simulink model "Casadi_Custom_Driver"  (R2016b)
settings: Solver=FixedStepDiscrete  StartTime=0.0  StopTime=inf  FixedStep=0.01  RelTol=1e-3  EnableMultiTasking=on
undefined symbols (not defined in the file): dimensionsFactor, DiscIntNeverNeededParam, vehicle_name, VehicleRoadInfoStructSize
libraries: simulink x39, SCANeR_API x36
(part 3 of 3)

== system Casadi_Custom_Driver/lateral control/Subsystem1/Enabled Subsystem1 ==
  In1 : Inport
  In2 : Inport  Port=2
  In3 : Inport  Port=3
  In4 : Inport  Port=4
  In5 : Inport  Port=5
  In6 : Inport  Port=6
  In7 : Inport  Port=7
  In8 : Inport  Port=8
  In9 : Inport  Port=9
  Enable : EnablePort
  MATLAB System6 : MATLABSystem  System=casadi_block_MPCtry_5  SimulateUsing=Interpreted execution
      mask Type: casadi_block_MPCtry_5
      mask Display:
      | disp('casadi_block_MPCtry_5');
      | port_label('input',1,'xd_in');
      | port_label('input',2,'yd_in');
      | port_label('input',3,'yawd_in');
      | port_label('input',4,'yaw_in');
      | port_label('input',5,'x_in');
      | port_label('input',6,'y_in');
      | port_label('input',7,'t');
      | port_label('input',8,'r');
      | port_label('input',9,'ex');
      | port_label('output',1,'delta_out');
      | port_label('output',2,'acc_out');
      | port_label('output',3,'break_out');
      | port_label('output',4,'vref');
      | port_label('output',5,'err');
  Out1 : Outport
  Out2 : Outport  Port=2
  Out3 : Outport  Port=3
  Out4 : Outport  Port=4
  Out5 : Outport  Port=5
  wires:
  In8/1 -> MATLAB System6/8
  MATLAB System6/1 -> Out1/1
  MATLAB System6/2 -> Out2/1
  MATLAB System6/3 -> Out3/1
  MATLAB System6/4 -> Out4/1
  MATLAB System6/5 -> Out5/1
  In1/1 -> MATLAB System6/1
  In2/1 -> MATLAB System6/2
  In3/1 -> MATLAB System6/3
  In4/1 -> MATLAB System6/4
  In5/1 -> MATLAB System6/5
  In6/1 -> MATLAB System6/6
  In7/1 -> MATLAB System6/7
  In9/1 -> MATLAB System6/9

== system Casadi_Custom_Driver/lateral control/Subsystem1/Enabled Subsystem2 ==
  In1 : Inport
  In2 : Inport  Port=2
  In3 : Inport  Port=3
  In4 : Inport  Port=4
  In5 : Inport  Port=5
  In6 : Inport  Port=6
  In7 : Inport  Port=7
  In8 : Inport  Port=8
  In9 : Inport  Port=9
  Enable : EnablePort
  MATLAB System : MATLABSystem  System=casadi_block_MPC_left_turn_onthego  SimulateUsing=Interpreted execution
      mask Type: casadi_block_MPC_left_turn_onthego
      mask Display:
      | disp('casadi_block_MPC_left_turn_onthego');
      | port_label('input',1,'xd_in');
      | port_label('input',2,'yd_in');
      | port_label('input',3,'yawd_in');
      | port_label('input',4,'yaw_in');
      | port_label('input',5,'x_in');
      | port_label('input',6,'y_in');
      | port_label('input',7,'t');
      | port_label('input',8,'r');
      | port_label('input',9,'alpha');
      | port_label('output',1,'delta_out');
      | port_label('output',2,'acc_out');
      | port_label('output',3,'break_out');
      | port_label('output',4,'vref');
      | port_label('output',5,'err');
  Out1 : Outport
  Out2 : Outport  Port=2
  Out3 : Outport  Port=3
  Out4 : Outport  Port=4
  Out5 : Outport  Port=5
  wires:
  In1/1 -> MATLAB System/1
  In2/1 -> MATLAB System/2
  In3/1 -> MATLAB System/3
  In4/1 -> MATLAB System/4
  In5/1 -> MATLAB System/5
  In7/1 -> MATLAB System/7
  In6/1 -> MATLAB System/6
  In9/1 -> MATLAB System/9
  In8/1 -> MATLAB System/8
  MATLAB System/1 -> Out1/1
  MATLAB System/2 -> Out2/1
  MATLAB System/3 -> Out3/1
  MATLAB System/4 -> Out4/1
  MATLAB System/5 -> Out5/1

== system Casadi_Custom_Driver/lateral control/Subsystem1/Enabled Subsystem3 ==
  In1 : Inport
  In2 : Inport  Port=2
  In3 : Inport  Port=3
  In4 : Inport  Port=4
  In5 : Inport  Port=5
  In6 : Inport  Port=6
  In7 : Inport  Port=7
  In8 : Inport  Port=8
  In9 : Inport  Port=9
  In10 : Inport  Port=10
  Enable : EnablePort
  MATLAB System : MATLABSystem  System=casadi_block_MPC_LSS_curve_onthego  SimulateUsing=Interpreted execution
      mask Type: casadi_block_MPC_LSS_curve_onthego
      mask Display:
      | disp('casadi_block_MPC_LSS_curve_onthego');
      | port_label('input',1,'xd_in');
      | port_label('input',2,'yd_in');
      | port_label('input',3,'yawd_in');
      | port_label('input',4,'yaw_in');
      | port_label('input',5,'x_in');
      | port_label('input',6,'y_in');
      | port_label('input',7,'t');
      | port_label('input',8,'R');
      | port_label('input',9,'vlat_ref');
      | port_label('input',10,'vlongi_ref');
      | port_label('output',1,'delta_out');
      | port_label('output',2,'acc_out');
      | port_label('output',3,'break_out');
      | port_label('output',4,'vref');
      | port_label('output',5,'err');
  Out1 : Outport
  Out2 : Outport  Port=2
  Out3 : Outport  Port=3
  Out4 : Outport  Port=4
  Out5 : Outport  Port=5
  wires:
  In1/1 -> MATLAB System/1
  In2/1 -> MATLAB System/2
  In3/1 -> MATLAB System/3
  In4/1 -> MATLAB System/4
  In5/1 -> MATLAB System/5
  In7/1 -> MATLAB System/7
  In6/1 -> MATLAB System/6
  MATLAB System/1 -> Out1/1
  MATLAB System/2 -> Out2/1
  MATLAB System/3 -> Out3/1
  MATLAB System/4 -> Out4/1
  MATLAB System/5 -> Out5/1
  In10/1 -> MATLAB System/10
  In9/1 -> MATLAB System/9
  In8/1 -> MATLAB System/8

== system Casadi_Custom_Driver/lateral control/Subsystem1/derivation ==
  note: Bricolage perso - a retester - 09/2019
  In1 : Inport
  Add : Sum  Inputs=+-
  Delay : Delay  DelayLength=10  SampleTime=0.01
  Discrete Derivative : simulink/Discrete/Discrete Derivative  gainval=1.0  ICPrevScaledInput=0.0  OutMin=[]  OutMax=[]  OutDataType=fixdt(1, 16)  OutScaling=2^-10  DoSatur=off
  Manual Switch : ManualSwitch
  Transfer Fcn First Order : simulink/Discrete/Transfer Fcn First Order  Commented=through  PoleZ=0.95  ICPrevOutput=0.0  DoSatur=off
  change_sign : Gain  Commented=through  Gain=-1
  coef : Gain  Gain=10
  Out1 : Outport
  wires:
  change_sign/1 -> Manual Switch/1
  coef/1 -> Transfer Fcn First Order/1
  Delay/1 -> Add/2
  Transfer Fcn First Order/1 -> change_sign/1
  In1/1 -> Discrete Derivative/1, Delay/1, Add/1
  Add/1 -> coef/1
  Discrete Derivative/1 -> Manual Switch/2
  Manual Switch/1 -> Out1/1

== system Casadi_Custom_Driver/lateral control/main lateral block/PI controller ==
  In1 : Inport
  Enable1 : EnablePort  StatesWhenEnabling=reset
  Discrete PID Controller3 : simulink/Continuous/PID Controller  Controller=PI  TimeDomain=Discrete-time  SampleTime=0.01  IntegratorMethod=Forward Euler  FilterMethod=Forward Euler  Form=Parallel  UseFilter=on  ControllerParametersSource=internal  P=1  I=0.4  D=1  N=1  InitialConditionSource=internal  InitialConditionForIntegrator=0  InitialConditionForFilter=0  ExternalReset=none  LimitOutput=off  UpperSaturationLimit=inf  LowerSaturationLimit=-inf  LinearizeAsGain=off  AntiWindupMode=none  Kb=1  TrackingMode=off  Kt=1  PParamMin=[]  PParamMax=[]  IParamMin=[]  IParamMax=[]  DParamMin=[]  DParamMax=[]  NParamMin=[]  NParamMax=[]  KbParamMin=[]  KbParamMax=[]  KtParamMin=[]  KtParamMax=[]  POutMin=[]  POutMax=[]  IOutMin=[]  IOutMax=[]  DOutMin=[]  DOutMax=[]  NOutMin=[]  NOutMax=[]  KbOutMin=[]  KbOutMax=[]  KtOutMin=[]  KtOutMax=[]  IntegratorOutMin=[]  IntegratorOutMax=[]  FilterOutMin=[]  FilterOutMax=[]  SumOutMin=[]  SumOutMax=[]  SumI1OutMin=[]  SumI1OutMax=[]  SumI2OutMin=[]  SumI2OutMax=[]  SumI3OutMin=[]  SumI3OutMax=[]  SumDOutMin=[]  SumDOutMax=[]  SaturationOutMin=[]  SaturationOutMax=[]  IntegratorContinuousStateAttributes=''  IntegratorStateMustResolveToSignalObject=off  IntegratorRTWStateStorageClass=Auto  FilterContinuousStateAttributes=''  FilterStateMustResolveToSignalObject=off  FilterRTWStateStorageClass=Auto  DifferentiatorICPrevScaledInput=0  DifferentiatorOutMin=[]  DifferentiatorOutMax=[]
  Out1 : Outport
  wires:
  Discrete PID Controller3/1 -> Out1/1
  In1/1 -> Discrete PID Controller3/1

== system Casadi_Custom_Driver/lateral control/main lateral block/Saturation ==
  Vh_Speed_kmh : Inport
  Steering_wheel_rad : Inport  Port=2
  Add5 : Sum  Inputs=+-  SampleTime=0.01
  Compare To Constant2 : simulink/Logic and Bit Operations/Compare To Constant  relop===  const=0  OutDataTypeStr=boolean
  Constant1 : Constant  Value=0
  Delay2 : Delay  DelayLength=1
  Gain1 : Gain  Gain=-1
  Mux1 : Mux  Inputs=2
  Saturation Dynamic : simulink/Discontinuities/Saturation Dynamic  OutMin=[]  OutMax=[]  OutDataTypeStr=Inherit: Same as second input  OutDataType=fixdt(1, 16)  OutScaling=2^-10  DoSatur=off
  Saturation acording vehicle speed : Lookup_n-D  NumberOfTableDimensions=1  BreakpointsForDimension1=[0,10,50,100,150]  BreakpointsForDimension1Min=0  BreakpointsForDimension1Max=150  Table=[1.3,1.25,1.1,0.8,0.3]  TableMin=0  TableMax=7.1  ExtrapMethod=Clip  UseLastTableValue=on  SampleTime=0.01  RndMeth=Simplest  InputSameDT=on
      settings: AttributesFormatString=%<Description>
  PID_sat_flag : Outport
  Driver_Action_to_SCANeR_Lat : Outport  Port=2
  wires:
  Gain1/1 -> Saturation Dynamic/3
  Saturation acording vehicle speed/1 -> Saturation Dynamic/1, Gain1/1
  Constant1/1 -> Mux1/2
  Steering_wheel_rad/1 -> Add5/1, Saturation Dynamic/2
  Add5/1 -> Delay2/1
  Compare To Constant2/1 -> PID_sat_flag/1
  Delay2/1 -> Compare To Constant2/1
  Mux1/1 -> Driver_Action_to_SCANeR_Lat/1
  Saturation Dynamic/1 -> Mux1/1, Add5/2
  Vh_Speed_kmh/1 -> Saturation acording vehicle speed/1

== system Casadi_Custom_Driver/lateral control/main lateral block/ShiftToGap ==
  note: z019013 :LAne gap part can be cleaned up
  note: This block allows to always output a required gap in meters, whatever may be the choice of shift type (1= meters / 0= lanes)
  note: z019013 : Added to v7p7p0 : to enable driver to maintian
      | lane center when offset of 0 is used
  Lane_gap_m : Inport
  Shift_Value : Inport  Port=2
  Shift_Type_1Met_0Lan : Inport  Port=3
  Compare To Constant : simulink/Logic and Bit Operations/Compare To Constant  relop=~=  const=0  OutDataTypeStr=boolean
  Constant : Constant
  Constant2 : Constant
  Logical Operator : Logic  Operator=OR  AllPortsSameDT=off  OutDataTypeStr=boolean
  Memory1 : Memory
  Product6 : Product  SampleTime=0.01  RndMeth=Zero
  Relational Operator : RelationalOperator  Operator===  OutDataTypeStr=boolean  RndMeth=Simplest
  Subsystem4 : Subsystem
  Switch1 : Switch  Criteria=u2 > Threshold  Threshold=0.5
  Switch3 : Switch  Criteria=u2 > Threshold  Threshold=0.5
  Lateral_Shift_flag : Outport
  Desired_Gap_offset_m : Outport  Port=2
  wires:
  Shift_Type_1Met_0Lan/1 -> Relational Operator/1, Switch1/2
  Product6/1 -> Switch1/3
  Lane_gap_m/1 -> Subsystem4/1(Lane_Gap_m)
  Switch1/1 -> Desired_Gap_offset_m/1
  Subsystem4/1(Lane_with_m) -> Product6/2
  Switch3/1 -> Logical Operator/1, Memory1/1
  Constant2/1 -> Switch3/1
  Memory1/1 -> Switch3/3
  Shift_Value/1 -> Compare To Constant/1, Switch1/1, Product6/1
  Compare To Constant/1 -> Switch3/2
  Relational Operator/1 -> Logical Operator/2
  Logical Operator/1 -> Lateral_Shift_flag/1
  Constant/1 -> Relational Operator/2

== system Casadi_Custom_Driver/lateral control/main lateral block/Subsystem ==
  Vehicle_Heading_rad : Inport
  Road_Angle_rad : Inport  Port=2
  Add5 : Sum  Inputs=+-  SampleTime=0.01
  Add6 : Sum  SampleTime=0.01
  Compare To Zero1 : simulink/Logic and Bit Operations/Compare To Zero  relop=>  OutDataTypeStr=boolean
  Constant3 : Constant
  Constant4 : Constant  Value=-1
  Product3 : Product  SampleTime=0.01  RndMeth=Zero
  Product4 : Product  SampleTime=0.01  RndMeth=Zero
  Switch1 : Switch  Threshold=0.5
  Trigonometric Function1 : Trigonometry
  Trigonometric Function2 : Trigonometry  Operator=cos
  Trigonometric Function3 : Trigonometry  Operator=cos
  Trigonometric Function4 : Trigonometry
  Vehicle_direction : Outport
  wires:
  Trigonometric Function1/1 -> Product3/1
  Trigonometric Function4/1 -> Product3/2
  Trigonometric Function2/1 -> Product4/1
  Trigonometric Function3/1 -> Product4/2
  Product3/1 -> Add6/1
  Product4/1 -> Add6/2
  Add6/1 -> Compare To Zero1/1
  Compare To Zero1/1 -> Switch1/2
  Constant4/1 -> Switch1/1
  Constant3/1 -> Switch1/3
  Switch1/1 -> Vehicle_direction/1
  Vehicle_Heading_rad/1 -> Add5/1, Trigonometric Function1/1, Trigonometric Function2/1
  Add5/1 -> Trigonometric Function3/1, Trigonometric Function4/1
  Road_Angle_rad/1 -> Add5/2

== system Casadi_Custom_Driver/lateral control/main lateral block/Subsystem1 ==
  Gap_offset_m : Inport
  Time_Gap_offset_s : Inport  Port=2
  Vh_Speed_kmh : Inport  Port=3
  Abs : Abs
  Add7 : Sum  Inputs=+-  SampleTime=0.01
  Constant : Constant  Value=-1
  Detect Change : simulink/Logic and Bit Operations/Detect Change  vinit=0  OutDataTypeStr=boolean
  Detect Change1 : simulink/Logic and Bit Operations/Detect Change  vinit=0  OutDataTypeStr=boolean
  Logical Operator : Logic  Operator=OR  AllPortsSameDT=off  OutDataTypeStr=boolean
  Manual Switch : ManualSwitch
  Product1 : Product  Inputs=*/  SampleTime=0.01  RndMeth=Zero
  Product2 : Product  Inputs=**  SampleTime=0.01  RndMeth=Zero
  Rate Limiter Dynamic : simulink/Discontinuities/Rate Limiter Dynamic
  Saturation : Saturate  UpperLimit=inf  LowerLimit=0
  Switch1 : Switch  Threshold=0.0
  Switch2 : Switch  Threshold=0.0
  Triggered Subsystem1 : Subsystem  TreatAsAtomicUnit=on
  coefficient acording vehicle speed1 : Lookup_n-D  NumberOfTableDimensions=1  BreakpointsForDimension1=[0,20,100,200]  Table=[3,3,1,1]  SampleTime=0.01  RndMeth=Simplest  InputSameDT=on
  lo : Constant  Value=-1
  lo1 : Constant
  Gap_offset_Final_m : Outport
  wires:
  Time_Gap_offset_s/1 -> Detect Change1/1, Add7/1
  coefficient acording vehicle speed1/1 -> Add7/2
  Add7/1 -> Saturation/1
  Vh_Speed_kmh/1 -> coefficient acording vehicle speed1/1
  Saturation/1 -> Product1/2
  [Gap_offset_m] -> Rate Limiter Dynamic/2, Switch1/2, Switch2/2
  lo/1 -> Switch1/1
  Rate Limiter Dynamic/1 -> Gap_offset_Final_m/1
  lo1/1 -> Switch2/3
  Gap_offset_m/1 -> Triggered Subsystem1/1(In1), Manual Switch/2, Abs/1, Detect Change/1
  Detect Change/1 -> Logical Operator/1
  Triggered Subsystem1/1(Out1) -> Manual Switch/1
  Manual Switch/1 -> [Gap_offset_m]
  Abs/1 -> Product1/1
  Product1/1 -> Product2/1, Switch2/1
  Product2/1 -> Switch1/3
  Constant/1 -> Product2/2
  Switch2/1 -> Rate Limiter Dynamic/1
  Switch1/1 -> Rate Limiter Dynamic/3
  Detect Change1/1 -> Logical Operator/2
  Logical Operator/1 -> Triggered Subsystem1/Trigger

== system Casadi_Custom_Driver/lateral control/main lateral block/Subsystem5 ==
  Road_Gap_m : Inport
  Road_Gap_Offset_m : Inport  Port=2
  Add5 : Sum  Inputs=+-  SampleTime=0.01
  Road_Gap_Err_m : Outport
  wires:
  Add5/1 -> Road_Gap_Err_m/1
  Road_Gap_m/1 -> Add5/2
  Road_Gap_Offset_m/1 -> Add5/1

== system Casadi_Custom_Driver/longitudinal control/Speed_Regulation/tolerance_calculation ==
  Cste2 : Constant  Value=vehicle_name  SampleTime=0.01
  Cste4 : Constant  Value=21  SampleTime=0.01
  Cste5 : Constant  Value=0.4  SampleTime=0.01
  Cste6 : Constant  Value=0.1  SampleTime=0.01
  Relational Operator : RelationalOperator  Operator===  OutDataTypeStr=boolean  RndMeth=Simplest
  Switch : Switch  Criteria=u2 > Threshold  Threshold=0.5
  Out1 : Outport
  wires:
  Switch/1 -> Out1/1
  Cste6/1 -> Switch/3
  Cste5/1 -> Switch/1
  Cste2/1 -> Relational Operator/1
  Cste4/1 -> Relational Operator/2
  Relational Operator/1 -> Switch/2

== system Casadi_Custom_Driver/Input_Signals_Management/Subsystem2/Road_Gap_Offset_Calculate1/Triggered Subsystem ==
  In1 : Inport
  Trigger : TriggerPort  VariantControl=Variant
  Out1 : Outport
  wires:
  In1/1 -> Out1/1

== system Casadi_Custom_Driver/lateral control/main lateral block/ShiftToGap/Subsystem4 ==
  Lane_Gap_m : Inport
  Subsystem3 : Subsystem
  Lane_with_m : Outport
  wires:
  Subsystem3/1(Lane_with_m) -> Lane_with_m/1
  Lane_Gap_m/1 -> Subsystem3/1(Lane_Gap_m)

== system Casadi_Custom_Driver/lateral control/main lateral block/Subsystem1/Triggered Subsystem1 ==
  In1 : Inport
  Trigger : TriggerPort  VariantControl=Variant
  Add : Sum
  Constant : Constant  Value=0
  Switch : Switch  Criteria=u2 ~= 0  Threshold=0.0
  Unit Delay : UnitDelay  SampleTime=-1
  Out1 : Outport
  wires:
  Unit Delay/1 -> Add/2
  Add/1 -> Switch/1, Switch/2, Unit Delay/1
  In1/1 -> Add/1
  Switch/1 -> Out1/1
  Constant/1 -> Switch/3

== system Casadi_Custom_Driver/lateral control/main lateral block/ShiftToGap/Subsystem4/Subsystem3 ==
  Lane_Gap_m : Inport
  Abs : Abs
  Abs1 : Abs
  Compare To Constant1 : simulink/Logic and Bit Operations/Compare To Constant  relop=>  const=1  OutDataTypeStr=boolean
  Compare To Zero : simulink/Logic and Bit Operations/Compare To Zero  relop=<  OutDataTypeStr=boolean
  Constant1 : Constant  Value=3.5
  Constant2 : Constant
  Logical Operator : Logic  AllPortsSameDT=off  OutDataTypeStr=boolean
  Logical Operator1 : Logic  Operator=NOT  AllPortsSameDT=off  OutDataTypeStr=boolean
  Memory : Memory
  Memory1 : Memory
  Product11 : Product
  Switch1 : Switch  Criteria=u2 > Threshold  Threshold=0.5
  Switch2 : Switch  Criteria=u2 > Threshold  Threshold=0.5
  Switch3 : Switch  Criteria=u2 > Threshold  Threshold=0.5
  Unit Delay : UnitDelay  SampleTime=-1
  g : Gain  Gain=2
  Lane_with_m : Outport
  wires:
  Switch3/1 -> Switch1/2, Memory1/1, Logical Operator1/1
  Lane_Gap_m/1 -> Unit Delay/1, Abs/1, Product11/1
  Constant2/1 -> Switch3/1
  Memory1/1 -> Switch3/3
  Compare To Constant1/1 -> Logical Operator/1
  Logical Operator/1 -> Switch3/2
  Switch1/1 -> g/1, Memory/1
  Memory/1 -> Switch1/1
  Product11/1 -> Compare To Zero/1
  Unit Delay/1 -> Product11/2, Switch1/3
  Compare To Zero/1 -> Logical Operator/2
  Abs/1 -> Compare To Constant1/1
  Switch2/1 -> Lane_with_m/1
  g/1 -> Abs1/1
  Constant1/1 -> Switch2/1
  Logical Operator1/1 -> Switch2/2
  Abs1/1 -> Switch2/3

== stateflow chart Casadi_Custom_Driver/longitudinal control/Accel_Regulation/Chart1 ==
  state Accel_Control/
    state Control_Off/
      accel_order= 0;
      brake_order= 0;
      accel_dyn= 0;
      brake_dyn= 0;
      int_epsilon = 0;
      Gear=10;
    state Controller/
      limit_accel = 1/kp_acc;
      limit_brake = 1/kp_brk;
      state Acceleration_regulation/
        state accel/
          control_state = 2;
          accel_order=1;
          brake_order= 0;
          accel_dyn=  kp_acc*epsilon + ki_acc*int_epsilon;
          brake_dyn= 0;
          Gear=10;
        (junction 59) -> accel [order 1] : [abs(epsilon) < limit_accel & control_state == 2]
            | {int_epsilon = int_epsilon + step_size*epsilon;}
        (junction 59) -> accel [order 2] : {int_epsilon = 0;}
      state Brake_regulation/
        state brake/
          control_state = 1;
          accel_order=0;
          brake_order=1;
          accel_dyn= 0;
          brake_dyn=  kp_brk*epsilon + ki_brk*int_epsilon;
          Gear=10;
        (junction 101) -> brake [order 1] : [abs(epsilon) < limit_brake & control_state == 1]
            | {int_epsilon = int_epsilon + step_size*epsilon;}
        (junction 101) -> brake [order 2] : {int_epsilon = 0;}
      accel -> (junction 56)
      brake -> (junction 56)
      (junction 56) -> (junction 59) [order 1] : [Accel_SP >= 0]
          | {epsilon =Accel_SP-Accel_Actual;}
      (junction 56) -> (junction 101) [order 2] : {epsilon =Accel_Actual-Accel_SP;}
    (default) -> (junction 55)
    (junction 55) -> Control_Off [order 1] : [Accel_control_on == 0]
    Control_Off -> (junction 55)
    Controller -> (junction 55) : [Accel_control_on == 0]
    (junction 55) -> (junction 56) [order 2] : {control_state = 0;}
  data: Accel_Actual input double; Accel_SP input double; Accel_control_on input double; accel_order output double; accel_dyn output double; brake_order output double; brake_dyn output double; kp_acc input double; ki_acc input double; kp_brk input double; ki_brk input double; step_size input double; limit_accel local double; limit_brake local double; epsilon output double; int_epsilon output double; control_state output double; Gear output double

== stateflow chart Casadi_Custom_Driver/longitudinal control/Speed_Regulation/Chart1 ==
  state Speed_Control/
    state Control_Off/
      accel = 0;
      brake = 0;
      int_epsilon = 0;
      Gear=3;
    state Controller/
      limit_accel = 1/kp_acc;
      limit_brake = 1/kp_brk;
      state normal_regulation/
        state normal_accel/
          control_state = 2;
          accel = -kp_acc*epsilon - ki_acc*int_epsilon;
          brake = 0;
          Gear_d = Gear;
        state normal_brake/
          control_state = 1;
          brake = kp_brk*epsilon + ki_brk*int_epsilon;
          accel = 0;
          Gear_d = Gear;
        (junction 58) -> (junction 59) [order 1] : [epsilon <= tolerance]
        (junction 58) -> (junction 57) [order 2]
        (junction 59) -> Speed_Control.Controller.normal_regulation.normal_accel [order 1] : [abs(epsilon) < limit_accel & control_state == 2]
            | {int_epsilon = int_epsilon + step_size*epsilon;}
        (junction 59) -> Speed_Control.Controller.normal_regulation.normal_accel [order 2] : {int_epsilon = 0;}
        (junction 57) -> Speed_Control.Controller.normal_regulation.normal_brake [order 1] : [abs(epsilon) < limit_brake & control_state == 1]
            | {int_epsilon = int_epsilon + step_size*epsilon;}
        (junction 57) -> Speed_Control.Controller.normal_regulation.normal_brake [order 2] : {int_epsilon = 0;}
        Speed_Control.Controller.normal_regulation.normal_brake -> (junction 69)
        Speed_Control.Controller.normal_regulation.normal_accel -> (junction 69)
      state reverse_regulation1/
        state normal_accel/
          control_state = 2;
          accel = -kp_acc*epsilon - ki_acc*int_epsilon;
          brake = 0;
          Gear_d = Gear;
        state normal_brake/
          control_state = 1;
          brake = kp_brk*epsilon + ki_brk*int_epsilon;
          accel = 0;
          Gear_d = Gear;
        (junction 123) -> (junction 124) [order 1] : [epsilon <=-0.1]
        (junction 123) -> (junction 125) [order 2]
        (junction 124) -> Speed_Control.Controller.reverse_regulation1.normal_accel [order 1] : [abs(epsilon) < limit_accel & control_state == 2]
            | {int_epsilon = int_epsilon + step_size*epsilon;}
        (junction 124) -> Speed_Control.Controller.reverse_regulation1.normal_accel [order 2] : {int_epsilon = 0;}
        (junction 125) -> Speed_Control.Controller.reverse_regulation1.normal_brake [order 1] : [abs(epsilon) < limit_brake & control_state == 1]
            | {int_epsilon = int_epsilon + step_size*epsilon;}
        (junction 125) -> Speed_Control.Controller.reverse_regulation1.normal_brake [order 2] : {int_epsilon = 0;}
        Speed_Control.Controller.reverse_regulation1.normal_brake -> (junction 126)
        Speed_Control.Controller.reverse_regulation1.normal_accel -> (junction 126)
      (junction 56) -> (junction 99) [order 1] : [setpoint< 0]
          | {epsilon =- speed+setpoint;}
      (junction 56) -> (junction 62) [order 2] : {epsilon = speed-setpoint;}
      (junction 62) -> (junction 58) : {Gear =10;}
      (junction 69) -> (junction 56)
      (junction 126) -> (junction 56)
      (junction 99) -> (junction 123) : {Gear =2;}
    (default) -> (junction 55)
    (junction 55) -> Control_Off [order 1] : [speed_control_on == 0]
    Control_Off -> (junction 55)
    Controller -> (junction 55) : [speed_control_on == 0]
    (junction 55) -> (junction 56) [order 2] : {control_state = 0;}
  data: speed input double; setpoint input double; speed_control_on input double; accel output double; brake output double; kp_acc input double; ki_acc input double; kp_brk input double; ki_brk input double; step_size input double; limit_accel local double; limit_brake local double; epsilon output double; int_epsilon output double; control_state output double; Gear_d output double; Gear local double; tolerance input double

== matlab function Casadi_Custom_Driver/longitudinal control/Speed_Regulation/MATLAB Function ==
  data: vehicle_name input; Kp_Accl output; Ki_Accl output; Intended_Vehicle_Speed_kmph input
function [Kp_Accl, Ki_Accl]= fcn(vehicle_name,Intended_Vehicle_Speed_kmph)
% This function calculates the Kp_Accl and Ki_Accl
% Following are the vehicle models to be used for simulation
% Vehicle_name:
% 0 = HHN
% 1 = BCB
% 2 = FFK
% 3 = KFKL1
% 4 = KFKL2
% 5 = KFKL1_VODM_CD04
% 6= KFKL1_VODM_CD05
% 7 = KFKL1_VODM_CD06
% 8 = FFKL1_VODM_CD06
% 9 = FFKL1_MMAC_CD06
% 10 = FFKL2_MMAC_CD06
% 11 = KFKL2_MMAC_CD06
% 12 = XDD

if (vehicle_name == 0)
    Kp_Accl = 0.3;
    Ki_Accl = 0.05;
elseif (vehicle_name == 1)
    Kp_Accl = 0.3;
    Ki_Accl = 0.05;
elseif (vehicle_name == 2)
    Kp_Accl = 0.1;
    Ki_Accl = 0.02;
elseif (vehicle_name == 3)
    Kp_Accl = 0.3;
    Ki_Accl = 0.02;
elseif (vehicle_name == 4)
    Kp_Accl = 0.3;
    Ki_Accl = 0.02;
elseif (vehicle_name == 5)
    Kp_Accl = 0.3;
    Ki_Accl = 0.02;
elseif (vehicle_name == 6)
    Kp_Accl = 0.3;
    Ki_Accl = 0.02;
elseif (vehicle_name == 7)
    Kp_Accl = 0.3;
    Ki_Accl = 0.02;
elseif (vehicle_name == 8)
    Kp_Accl = 0.3;
    Ki_Accl = 0.02;
elseif (vehicle_name == 9)
    Kp_Accl = 0.3;
    Ki_Accl = 0.02;
elseif (vehicle_name == 10)
    Kp_Accl = 0.3;
    Ki_Accl = 0.02;
elseif (vehicle_name == 11)
    Kp_Accl = 0.3;
    Ki_Accl = 0.02;
elseif (vehicle_name == 17)% HCB 60kwh
    if Intended_Vehicle_Speed_kmph >= 60
        Kp_Accl = 0.3; %0.1
        Ki_Accl = 0.05;%0.01
    else
        Kp_Accl = 0.1; %0.1
        Ki_Accl = 0.01;%0.01
    end
elseif (vehicle_name == 13) || (vehicle_name == 15) % BCB
    Kp_Accl =0.3;
    Ki_Accl = 0.05;
elseif (vehicle_name == 18) || (vehicle_name == 14) || (vehicle_name == 12)% XDD vehicle
    Kp_Accl = 0.3;
    Ki_Accl = 0.05;
elseif (vehicle_name == 19)% BCB 40kwh Correl
    if Intended_Vehicle_Speed_kmph >= 50
        Kp_Accl = 1;
        Ki_Accl = 0.1;
    else
        Kp_Accl = 0.1; %0.1
        Ki_Accl = 0.01;%0.01
    end
elseif (vehicle_name == 16) % HHN Correl
    if Intended_Vehicle_Speed_kmph >= 15
        Kp_Accl = 0.3;
        Ki_Accl = 0.05;
    elseif Intended_Vehicle_Speed_kmph < 7
        Kp_Accl = 0.3;
        Ki_Accl = 0.05;
    else
        Kp_Accl = 0.009;
        Ki_Accl = 0.00032;
    end
elseif (vehicle_name == 20) % Echo
    Kp_Accl = 0.3;
    Ki_Accl = 0.05;
elseif (vehicle_name == 21) % Torque Management
    Kp_Accl = 0.0012;
    Ki_Accl = 0.0012;
else  % Other vehicles
    if Intended_Vehicle_Speed_kmph >= 15
        Kp_Accl = 0.3;
        Ki_Accl = 0.05;
    else
        Kp_Accl = 0.009;
        Ki_Accl = 0.00032;
    end
end

== stateflow chart Casadi_Custom_Driver/driver manager/Chart ==
  state Variablesetting
    entry:
    Driver_Action_to_SCANeR_Long;
    Driver_Action_to_SCANeR_Lat;
    Null_longitudinal;
    Null_lateral;
    manual_acc_brk;
    manual_acc_brk_val;
    APK_steer_rad;
    APK_steer_rad_val;
  state driverstatus0
    entry:
    longitudinal = Null_longitudinal;
    lateral = Null_lateral;
    if APK_steer_rad_val > 0
    lateral = APK_steer_rad;
    end
    if manual_acc_brk_val >0
    longitudinal = manual_acc_brk;
    end
  state driverstatus3
    entry:
    longitudinal = Driver_Action_to_SCANeR_Long;
    lateral = Null_lateral;
    if APK_steer_rad_val > 0
    lateral = APK_steer_rad;
    end
    if manual_acc_brk_val > 0
    longitudinal = manual_acc_brk;
    end
  state driverstatus2
    entry:
    longitudinal = Null_longitudinal;
    lateral = Driver_Action_to_SCANeR_Lat;
    if APK_steer_rad_val > 0
    lateral = APK_steer_rad;
    end
    if manual_acc_brk_val > 0
    longitudinal = manual_acc_brk;
    end
  state driverstatus1
    entry:
    longitudinal = Driver_Action_to_SCANeR_Long;
    lateral = Driver_Action_to_SCANeR_Lat;
    if APK_steer_rad_val > 0
    lateral = APK_steer_rad;
    end
    if manual_acc_brk_val > 0
    longitudinal = manual_acc_brk;
    end
  state driverstatus4
    entry:
    longitudinal = Temp_longitudinal_GLOSA;
    lateral = Temp_lateral_GLOSA;
    if APK_steer_rad_val > 0
    lateral = APK_steer_rad;
    end
    if manual_acc_brk_val > 0
    longitudinal = manual_acc_brk;
    end
  (default) -> Variablesetting
  Variablesetting -> (junction 29)
  driverstatus3 -> (junction 29)
  driverstatus0 -> (junction 29)
  (junction 29) -> driverstatus3 [order 5] : [Driver_status == 3]
  (junction 29) -> driverstatus0 [order 1] : [Driver_status == 0]
  (junction 29) -> driverstatus1 [order 2] : [Driver_status == 1 || Driver_status > 4]
  (junction 29) -> driverstatus2 [order 4] : [Driver_status == 2]
  driverstatus4 -> (junction 29)
  (junction 29) -> driverstatus4 [order 3] : [Driver_status == 4]
  driverstatus1 -> (junction 29)
  driverstatus2 -> (junction 29)
  data: Driver_Action_to_SCANeR_Long input; Driver_Action_to_SCANeR_Lat input; Null_longitudinal input; Null_lateral input; manual_acc_brk input; manual_acc_brk_val input; APK_steer_rad input; APK_steer_rad_val input; Driver_status input; lateral output; longitudinal output; Temp_longitudinal_GLOSA input; Temp_lateral_GLOSA input
